simulink model "fuzzy_simulink"  (R2019a)
settings: Solver=VariableStepAuto  StartTime=0.0  StopTime=10  RelTol=1e-3
libraries: fuzblock x1
settings Model: Creator=Afiff  LastModifiedBy=ancem
settings DataIOCC: ReturnWorkspaceOutputs=off
settings DebuggingCC: ArithmeticOperatorsInVariantConditions=warning
settings SFSimCC: SimUseLocalCustomCode=off
settings RTWCC: RTWUseLocalCustomCode=off
settings CodeAppCC: StateflowObjectComments=on

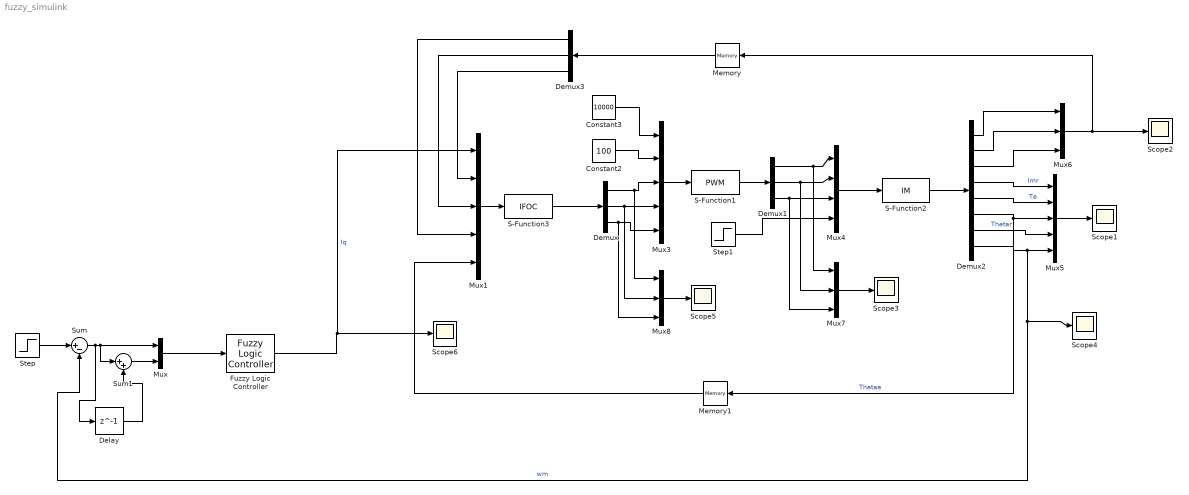
== system fuzzy_simulink ==
  Constant2 : Constant  Value=100
  Constant3 : Constant  Value=10000
  Delay : Delay  DelayLength=1  InitialCondition=0
  Demux : Demux  Outputs=3
  Demux1 : Demux  Outputs=3
  Demux2 : Demux  Outputs=8
  Demux3 : Demux  Outputs=3
  Fuzzy Logic Controller : fuzblock/Fuzzy Logic  Controller  FIS='fuzzys.fis'  OutputSampleNumber=101  DataType=double  FuzzifiedInputs=off  RuleFiringStrengths=off  RuleOutputs=off  AggregatedOutputs=off  SimulateUsing=Interpreted execution  OutOfRangeInputValueMessage=warning  NoRuleFiredMessage=warning  EmptyOutputFuzzySetMessage=warning
  Memory : Memory
  Memory1 : Memory
  Mux : Mux  Inputs=2
  Mux1 : Mux  Inputs=5
  Mux3 : Mux  Inputs=5
  Mux4 : Mux
  Mux5 : Mux  Inputs=5
  Mux6 : Mux  Inputs=3
  Mux7 : Mux  Inputs=3
  Mux8 : Mux  Inputs=3
  S-Function1 : S-Function  FunctionName=PWM  SFunctionModules='PWM'  SFunctionDeploymentMode=off  EnableBusSupport=off
  S-Function2 : S-Function  FunctionName=IM  SFunctionModules='IM'  SFunctionDeploymentMode=off  EnableBusSupport=off
  S-Function3 : S-Function  FunctionName=IFOC  SFunctionModules='IFOC'  SFunctionDeploymentMode=off  EnableBusSupport=off
  Scope{1..6} (6 alike) : Scope
  Step : Step  After=100  SampleTime=0
  Step1 : Step  Time=5  After=30  SampleTime=0
  Sum : Sum  Inputs=|+-
  Sum1 : Sum  Inputs=|++
  wires:
  S-Function3/1 -> Demux/1
  Mux3/1 -> S-Function1/1
  Demux/1 -> Mux8/1, Mux3/3
  Demux/2 -> Mux8/2, Mux3/4
  Constant3/1 -> Mux3/1
  Constant2/1 -> Mux3/2
  S-Function1/1 -> Demux1/1
  Demux1/1 -> Mux7/1, Mux4/1
  Demux1/2 -> Mux7/2, Mux4/2
  Demux1/3 -> Mux7/3, Mux4/3
  Step1/1 -> Mux4/4
  Mux4/1 -> S-Function2/1
  S-Function2/1 -> Demux2/1
  Demux2/7 -> Mux5/4  "Thetar"
  Demux2/6 -> Mux5/3, Memory1/1  "Thetae"
  Demux2/5 -> Mux5/2  "Te"
  Demux2/4 -> Mux5/1  "Imr"
  Demux2/3 -> Mux6/3
  Demux2/2 -> Mux6/2
  Demux2/1 -> Mux6/1
  Mux5/1 -> Scope1/1
  Mux6/1 -> Scope2/1, Memory/1
  Memory/1 -> Demux3/1
  Demux3/3 -> Mux1/2
  Mux7/1 -> Scope3/1
  Demux2/8 -> Scope4/1, Sum/2, Mux5/5  "wm"
  Mux8/1 -> Scope5/1
  Demux/3 -> Mux8/3, Mux3/5
  Fuzzy Logic Controller/1 -> Mux1/1, Scope6/1  "Iq"
  Mux/1 -> Fuzzy Logic Controller/1
  Step/1 -> Sum/1
  Sum/1 -> Delay/1, Sum1/1, Mux/1
  Sum1/1 -> Mux/2
  Delay/1 -> Sum1/2
  Mux1/1 -> S-Function3/1
  Demux3/2 -> Mux1/3
  Demux3/1 -> Mux1/4
  Memory1/1 -> Mux1/5
